simulink model "updated_target_driver_2026_withVariants_MPC_andwlqp"  (R2024b)
settings: Solver=FixedStepDiscrete  StartTime=0.0  StopTime=running_time  FixedStep=dt_s  RelTol=1e-3
values from neighbouring files (symbols this model uses):
  A = gamma_2*gamma_3*Thrust_desired    [force2voltage.m]
  a2_lb = -0.25    [target_driver_setup_2022_Ctrl_V_2_4.m]    (also in target_driver_setup_2022_Ctrl_V_2_4_geometric.m; target_driver_setup_mpc_12msdelay.m; target_driver_setup_mpc_andWLQP.m)
  a2_openloop = 0    [target_driver_setup_2022_Ctrl_V_2_4.m]    (also in target_driver_setup_2022_Ctrl_V_2_4_geometric.m; target_driver_setup_mpc_12msdelay.m; target_driver_setup_mpc_andWLQP.m)
  a2_ub = 0.25    [target_driver_setup_2022_Ctrl_V_2_4.m]    (also in target_driver_setup_2022_Ctrl_V_2_4_geometric.m; target_driver_setup_mpc_12msdelay.m; target_driver_setup_mpc_andWLQP.m)
  att_s = 500    [target_driver_setup_2022_Ctrl_V_2_4.m]    (also in target_driver_setup_2022_Ctrl_V_2_4_geometric.m; target_driver_setup_mpc_12msdelay.m; target_driver_setup_mpc_andWLQP.m)
  b_1_d_desired = [1,0,0]    [target_driver_setup_2022_Ctrl_V_2_4.m]    (also in target_driver_setup_2022_Ctrl_V_2_4_geometric.m; target_driver_setup_mpc_12msdelay.m; target_driver_setup_mpc_andWLQP.m)
  closedloop_flag = 0    [target_driver_setup_2022_Ctrl_V_2_4.m]    (also in target_driver_setup_2022_Ctrl_V_2_4_geometric.m; target_driver_setup_mpc_12msdelay.m; target_driver_setup_mpc_andWLQP.m)
  delay = delay-vicon_sample_cycle/2    [target_driver_setup_2022_Ctrl_V_2_4.m]    (also in target_driver_setup_2022_Ctrl_V_2_4_geometric.m; target_driver_setup_mpc_12msdelay.m; target_driver_setup_mpc_andWLQP.m)
  drv_amp = abs((vleft_p2p-vright_p2p))/2+min(vleft_p2p,vright_p2p)    [Wing_traj_to_Voltage.m]    (also in force2voltage.m; target_driver_setup_2022_Ctrl_V_2_4.m = 150; target_driver_setup_2022_Ctrl_V_2_4_geometric.m = 110; target_driver_setup_mpc_12msdelay.m = 150)
  drv_bias = max_drv_bias    (= 200)    [target_driver_setup_2022_Ctrl_V_2_4.m]    (also in target_driver_setup_2022_Ctrl_V_2_4_geometric.m; target_driver_setup_mpc_12msdelay.m; target_driver_setup_mpc_andWLQP.m)
  drv_pitch_left = vleft_pitch    [Wing_traj_to_Voltage.m]    (also in force2voltage.m = 0; target_driver_setup_2022_Ctrl_V_2_4.m = 9.05; target_driver_setup_2022_Ctrl_V_2_4_geometric.m = 9.05; target_driver_setup_mpc_12msdelay.m = 9.05)
  drv_pitch_right = vright_pitch    [Wing_traj_to_Voltage.m]    (also in force2voltage.m = 0; target_driver_setup_2022_Ctrl_V_2_4.m = 9.05; target_driver_setup_2022_Ctrl_V_2_4_geometric.m = 9.05; target_driver_setup_mpc_12msdelay.m = 9.05)
  drv_roll = (vleft_p2p-vright_p2p)/4    [Wing_traj_to_Voltage.m]    (also in force2voltage.m; target_driver_setup_2022_Ctrl_V_2_4.m = -0.001; target_driver_setup_2022_Ctrl_V_2_4_geometric.m = -0.001; target_driver_setup_mpc_12msdelay.m = -0.001)
  dt_s = 2.0e-4    (= 0.0002)    [target_driver_setup_2022_Ctrl_V_2_4.m]    (also in target_driver_setup_2022_Ctrl_V_2_4_geometric.m; target_driver_setup_mpc_12msdelay.m; target_driver_setup_mpc_andWLQP.m)
  f_fin = f    (= 155)    [target_driver_setup_2022_Ctrl_V_2_4.m]    (also in target_driver_setup_2022_Ctrl_V_2_4_geometric.m; target_driver_setup_mpc_12msdelay.m; target_driver_setup_mpc_andWLQP.m)
  f_int = f    (= 155)    [target_driver_setup_2022_Ctrl_V_2_4.m]    (also in target_driver_setup_2022_Ctrl_V_2_4_geometric.m; target_driver_setup_mpc_12msdelay.m; target_driver_setup_mpc_andWLQP.m)
  g = 9.8    [target_driver_setup_2022_Ctrl_V_2_4.m]    (also in target_driver_setup_2022_Ctrl_V_2_4_geometric.m; target_driver_setup_mpc_12msdelay.m; target_driver_setup_mpc_andWLQP.m; test_full_attitude_mpc.m = 9.81)
  I_moment_vec = [Ixx, Iyy, Izz]    [target_driver_setup_2022_Ctrl_V_2_4.m]    (also in target_driver_setup_2022_Ctrl_V_2_4_geometric.m; target_driver_setup_mpc_12msdelay.m; target_driver_setup_mpc_andWLQP.m)
  k_tau_vec = [k_tau_roll;k_tau_pitch]    [target_driver_setup_2022_Ctrl_V_2_4.m]    (also in target_driver_setup_2022_Ctrl_V_2_4_geometric.m; target_driver_setup_mpc_12msdelay.m; target_driver_setup_mpc_andWLQP.m)
  landing_flag = 0    [target_driver_setup_2022_Ctrl_V_2_4.m]    (also in target_driver_setup_2022_Ctrl_V_2_4_geometric.m; target_driver_setup_mpc_12msdelay.m; target_driver_setup_mpc_andWLQP.m)
  landing_parameter = [start_delay+T,transition_rate, rising_time, falling_time, landing_rising_time, landing_z_decrease, landing_y_decrease, landing_x_decrease]    [target_driver_setup_2022_Ctrl_V_2_4.m]    (also in target_driver_setup_2022_Ctrl_V_2_4_geometric.m; target_driver_setup_mpc_12msdelay.m; target_driver_setup_mpc_andWLQP.m)
  low_bound = -5    [target_driver_setup_2022_Ctrl_V_2_4.m]    (also in target_driver_setup_2022_Ctrl_V_2_4_geometric.m; target_driver_setup_mpc_12msdelay.m = -10; target_driver_setup_mpc_andWLQP.m = -10)
  low_bound_eR = -1.2    [target_driver_setup_2022_Ctrl_V_2_4.m]    (also in target_driver_setup_2022_Ctrl_V_2_4_geometric.m; target_driver_setup_mpc_12msdelay.m; target_driver_setup_mpc_andWLQP.m)
  low_bound_vx = -0.5    [target_driver_setup_2022_Ctrl_V_2_4.m]    (also in target_driver_setup_2022_Ctrl_V_2_4_geometric.m; target_driver_setup_mpc_12msdelay.m; target_driver_setup_mpc_andWLQP.m)
  low_bound_vy = -0.5    [target_driver_setup_2022_Ctrl_V_2_4.m]    (also in target_driver_setup_2022_Ctrl_V_2_4_geometric.m; target_driver_setup_mpc_12msdelay.m; target_driver_setup_mpc_andWLQP.m)
  low_bound_vz = -0.5    [target_driver_setup_2022_Ctrl_V_2_4.m]    (also in target_driver_setup_2022_Ctrl_V_2_4_geometric.m; target_driver_setup_mpc_12msdelay.m; target_driver_setup_mpc_andWLQP.m)
  low_bound_x = -0.1    [target_driver_setup_2022_Ctrl_V_2_4.m]    (also in target_driver_setup_2022_Ctrl_V_2_4_geometric.m; target_driver_setup_mpc_12msdelay.m = -0.6; target_driver_setup_mpc_andWLQP.m = -0.6)
  low_bound_y = -0.06    [target_driver_setup_2022_Ctrl_V_2_4.m]    (also in target_driver_setup_2022_Ctrl_V_2_4_geometric.m; target_driver_setup_mpc_12msdelay.m = -0.6; target_driver_setup_mpc_andWLQP.m = -0.6)
  low_bound_z = -0.04    [target_driver_setup_2022_Ctrl_V_2_4.m]    (also in target_driver_setup_2022_Ctrl_V_2_4_geometric.m; target_driver_setup_mpc_12msdelay.m = -0.1; target_driver_setup_mpc_andWLQP.m = -0.1)
  m = t <= t_zoom    [plot_roll_torque_cmd_vs_actual.m]    (also in plot_roll_torque_cmd_vs_actual_flightlog.m = t >= t0 & t <= t1; target_driver_setup_2022_Ctrl_V_2_4.m = 8.5655e-05; target_driver_setup_2022_Ctrl_V_2_4_geometric.m = 8.5655e-05; target_driver_setup_mpc_12msdelay.m = 8.5655e-05)
  params_vec = [params_opt.delta_1, params_opt.delta_2, params_opt.delta_3,      params_opt.gamma_1, params_opt.gamma_2_1, params_opt.gamma_3,      params_opt.eta, params_opt.nu, params_opt.mu]'    [force2voltage_tuningSandbox.m]    (also in target_driver_setup_2022_Ctrl_V_2_4.m = [params_opt.delta_1, params_opt.delta_2, params_opt.delta_3,; target_driver_setup_2022_Ctrl_V_2_4_geometric.m = [params_opt.delta_1, params_opt.delta_2, params_opt.delta_3,; target_driver_setup_mpc_12msdelay.m = [params_opt.delta_1, params_opt.delta_2, params_opt.delta_3,; target_driver_setup_mpc_andWLQP.m = [params_opt.delta_1, params_opt.delta_2, params_opt.delta_3,)
  phase = 0    [target_driver_setup_2022_Ctrl_V_2_4.m]    (also in target_driver_setup_2022_Ctrl_V_2_4_geometric.m; target_driver_setup_mpc_12msdelay.m; target_driver_setup_mpc_andWLQP.m)
  r_desired = [default_x, default_y,z_desired]    [target_driver_setup_2022_Ctrl_V_2_4.m]    (also in target_driver_setup_2022_Ctrl_V_2_4_geometric.m; target_driver_setup_mpc_12msdelay.m; target_driver_setup_mpc_andWLQP.m)
  roll_offset_angle = 0    [target_driver_setup_2022_Ctrl_V_2_4.m]    (also in target_driver_setup_2022_Ctrl_V_2_4_geometric.m; target_driver_setup_mpc_12msdelay.m; target_driver_setup_mpc_andWLQP.m)
  running_time = start_delay+T    (= 10)    [target_driver_setup_2022_Ctrl_V_2_4.m]    (also in target_driver_setup_2022_Ctrl_V_2_4_geometric.m; target_driver_setup_mpc_12msdelay.m = 0.5; target_driver_setup_mpc_andWLQP.m)
  running_time_control = start_delay_control+T+0.0    (= 10)    [target_driver_setup_2022_Ctrl_V_2_4.m]    (also in target_driver_setup_2022_Ctrl_V_2_4_geometric.m; target_driver_setup_mpc_12msdelay.m = 0.5; target_driver_setup_mpc_andWLQP.m)
  sampling_f = 1/dt_s    (= 5000)    [target_driver_setup_2022_Ctrl_V_2_4.m]    (also in target_driver_setup_2022_Ctrl_V_2_4_geometric.m; target_driver_setup_mpc_12msdelay.m; target_driver_setup_mpc_andWLQP.m)
  start_delay = 0.0    (= 0)    [target_driver_setup_2022_Ctrl_V_2_4.m]    (also in target_driver_setup_2022_Ctrl_V_2_4_geometric.m; target_driver_setup_mpc_12msdelay.m; target_driver_setup_mpc_andWLQP.m)
  start_delay_control = start_delay + ramp_delay    (= 0)    [target_driver_setup_2022_Ctrl_V_2_4.m]    (also in target_driver_setup_2022_Ctrl_V_2_4_geometric.m; target_driver_setup_mpc_12msdelay.m; target_driver_setup_mpc_andWLQP.m)
  T = 10    [target_driver_setup_2022_Ctrl_V_2_4.m]    (also in target_driver_setup_2022_Ctrl_V_2_4_geometric.m; target_driver_setup_mpc_12msdelay.m = 0.5; target_driver_setup_mpc_andWLQP.m; test_full_attitude_mpc.m = T0 + nu(1))
  task_flag = 0    [target_driver_setup_2022_Ctrl_V_2_4.m]    (also in target_driver_setup_2022_Ctrl_V_2_4_geometric.m; target_driver_setup_mpc_12msdelay.m; target_driver_setup_mpc_andWLQP.m)
  task_parameter = [radius_ref, frequency_ref, radius_ratio, lissajous_ratio, lissajous_delta, lissajous_amplitude_ratio,z_radius_ratio]    [target_driver_setup_2022_Ctrl_V_2_4.m]    (also in target_driver_setup_2022_Ctrl_V_2_4_geometric.m; target_driver_setup_mpc_12msdelay.m; target_driver_setup_mpc_andWLQP.m)
  upp_bound = 5    [target_driver_setup_2022_Ctrl_V_2_4.m]    (also in target_driver_setup_2022_Ctrl_V_2_4_geometric.m; target_driver_setup_mpc_12msdelay.m = 10; target_driver_setup_mpc_andWLQP.m = 10)
  upp_bound_eR = 1.2    [target_driver_setup_2022_Ctrl_V_2_4.m]    (also in target_driver_setup_2022_Ctrl_V_2_4_geometric.m; target_driver_setup_mpc_12msdelay.m; target_driver_setup_mpc_andWLQP.m)
  upp_bound_vx = 0.5    [target_driver_setup_2022_Ctrl_V_2_4.m]    (also in target_driver_setup_2022_Ctrl_V_2_4_geometric.m; target_driver_setup_mpc_12msdelay.m; target_driver_setup_mpc_andWLQP.m)
  upp_bound_vy = 0.5    [target_driver_setup_2022_Ctrl_V_2_4.m]    (also in target_driver_setup_2022_Ctrl_V_2_4_geometric.m; target_driver_setup_mpc_12msdelay.m; target_driver_setup_mpc_andWLQP.m)
  upp_bound_vz = 0.5    [target_driver_setup_2022_Ctrl_V_2_4.m]    (also in target_driver_setup_2022_Ctrl_V_2_4_geometric.m; target_driver_setup_mpc_12msdelay.m; target_driver_setup_mpc_andWLQP.m)
  upp_bound_x = 0.1    [target_driver_setup_2022_Ctrl_V_2_4.m]    (also in target_driver_setup_2022_Ctrl_V_2_4_geometric.m; target_driver_setup_mpc_12msdelay.m = 0.6; target_driver_setup_mpc_andWLQP.m = 0.6)
  upp_bound_y = 0.06    [target_driver_setup_2022_Ctrl_V_2_4.m]    (also in target_driver_setup_2022_Ctrl_V_2_4_geometric.m; target_driver_setup_mpc_12msdelay.m = 0.6; target_driver_setup_mpc_andWLQP.m = 0.6)
  upp_bound_z = 0.04    [target_driver_setup_2022_Ctrl_V_2_4.m]    (also in target_driver_setup_2022_Ctrl_V_2_4_geometric.m; target_driver_setup_mpc_12msdelay.m = 0.1; target_driver_setup_mpc_andWLQP.m = 0.1)
  weights_vec = [ws; wds; wpr_xy;wpr_z; wpf; wvr_xy; wvr_z ... (first row only)    [target_driver_setup_2022_Ctrl_V_2_4.m]    (also in target_driver_setup_2022_Ctrl_V_2_4_geometric.m; target_driver_setup_mpc_12msdelay.m; target_driver_setup_mpc_andWLQP.m)
undefined symbols (not defined in the file or in its folder): Com1, ctrl_Ts, DiscIntNeverNeededParam, dspblkCoreblockFVToolHelper, gcbh, left_mapping, left_mapping_F_to_Phi, lp_den, lp_num, none, right_mapping, right_mapping_F_to_Phi, vlp_den, vlp_num
libraries: simulink x18, xpcseriallib x2, cstblocks x1, xpcnilib x1, xpcutilitieslib x1
(part 2 of 6)

== system updated_target_driver_2026_withVariants_MPC_andwlqp/Variant Subsystem/Experimental ==
  EnableSignal : Inport
  frequency (hz) : Inport  Port=2
  Amplitude : Inport  Port=3
  PitchBias V (left) : Inport  Port=4
  RollBias V : Inport  Port=5
  PitchBias V (right) : Inport  Port=6
  a2 : Inport  Port=7
  Bias_v : Inport  Port=8
  Phase (deg) : Inport  Port=9
  In10 : Inport  Port=10
  PCI-6259 DA1 : xpcnilib/D//A/M Series/PCI-6259 DA  channel=[1:4]  range=[10,5, 10, 10]  reset=[1 1 1 1]  initValue=[0 0 0 0]  sampletime=-1  slot=-1
      settings: SourceProductName=Simulink Real-Time
  Vicon Measurements1 : Subsystem
  signal generator a3 : Subsystem
  bias2 : Outport
  LW signal : Outport  Port=2
  RW signal : Outport  Port=3
  X (m) : Outport  Port=4
  Y (m) : Outport  Port=5
  Z (m) : Outport  Port=6
  alpha (radians) : Outport  Port=7
  beta (radians) : Outport  Port=8
  gamma (radians) : Outport  Port=9
  wires:
  Vicon Measurements1/2(Y (m)) -> Y (m)/1
  PitchBias V (right)/1 -> signal generator a3/8(PitchBias V (right))
  a2/1 -> signal generator a3/9(a2)
  Phase (deg)/1 -> signal generator a3/7(Phase (deg))
  Vicon Measurements1/4(alpha (radians)) -> alpha (radians)/1
  frequency (hz)/1 -> signal generator a3/3(frequency (hz))
  RollBias V/1 -> signal generator a3/6(RollBias V)
  Bias_v/1 -> signal generator a3/2(Bias_v)
  Vicon Measurements1/6(gamma (radians)) -> gamma (radians)/1
  Amplitude/1 -> signal generator a3/4(Amplitude)
  Vicon Measurements1/5(beta (radians)) -> beta (radians)/1
  signal generator a3/3(D2A DriveSignal 2) -> RW signal/1, PCI-6259 DA1/3
  signal generator a3/1(Bias_D2A) -> bias2/1, PCI-6259 DA1/1
  Vicon Measurements1/1(X (m)) -> X (m)/1
  Vicon Measurements1/3(Z (m)) -> Z (m)/1
  In10/1 -> PCI-6259 DA1/4
  PitchBias V (left)/1 -> signal generator a3/5(PitchBias V (left))
  EnableSignal/1 -> signal generator a3/1(EnableSignal)
  signal generator a3/2(D2A DriveSignal 1) -> LW signal/1, PCI-6259 DA1/2

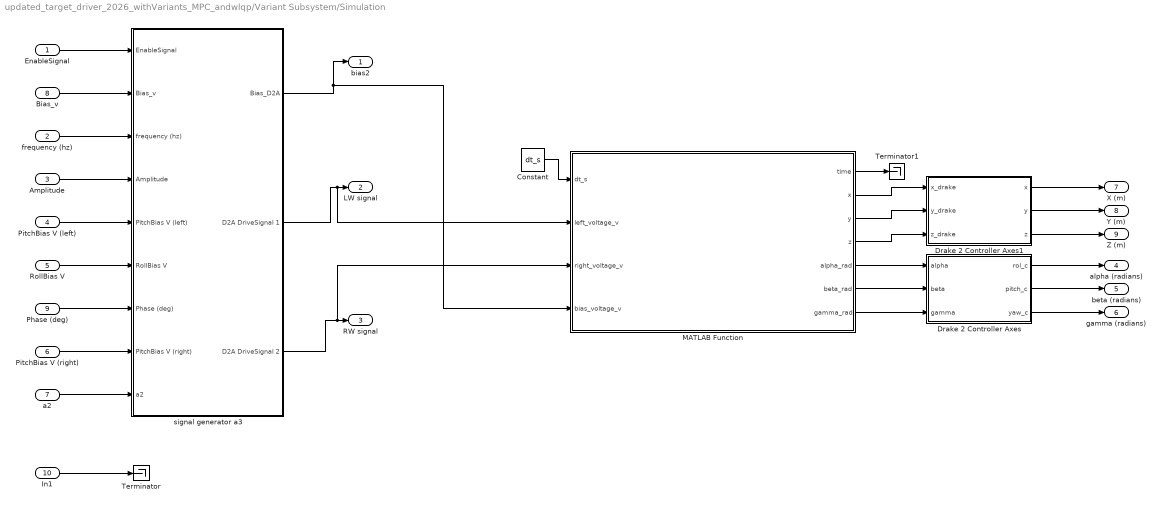
== system updated_target_driver_2026_withVariants_MPC_andwlqp/Variant Subsystem/Simulation ==
  EnableSignal : Inport
  frequency (hz) : Inport  Port=2
  Amplitude : Inport  Port=3
  PitchBias V (left) : Inport  Port=4
  RollBias V : Inport  Port=5
  PitchBias V (right) : Inport  Port=6
  a2 : Inport  Port=7
  Bias_v : Inport  Port=8
  Phase (deg) : Inport  Port=9
  In1 : Inport  Port=10
  Constant : Constant  Value=dt_s
  Drake 2 Controller Axes : MATLAB Function  TreatAsAtomicUnit=on
  Drake 2 Controller Axes1 : MATLAB Function  TreatAsAtomicUnit=on
  MATLAB Function : MATLAB Function  TreatAsAtomicUnit=on  VariantControl=Choice_1
  Terminator : Terminator
  Terminator1 : Terminator
  signal generator a3 : Subsystem
  bias2 : Outport
  LW signal : Outport  Port=2
  RW signal : Outport  Port=3
  alpha (radians) : Outport  Port=4
  beta (radians) : Outport  Port=5
  gamma (radians) : Outport  Port=6
  X (m) : Outport  Port=7
  Y (m) : Outport  Port=8
  Z (m) : Outport  Port=9
  wires:
  signal generator a3/1(Bias_D2A) -> bias2/1, MATLAB Function/4(bias_voltage_v)
  Constant/1 -> MATLAB Function/1(dt_s)
  signal generator a3/3(D2A DriveSignal 2) -> MATLAB Function/3(right_voltage_v), RW signal/1
  a2/1 -> signal generator a3/9(a2)
  PitchBias V (left)/1 -> signal generator a3/5(PitchBias V (left))
  Amplitude/1 -> signal generator a3/4(Amplitude)
  Bias_v/1 -> signal generator a3/2(Bias_v)
  PitchBias V (right)/1 -> signal generator a3/8(PitchBias V (right))
  RollBias V/1 -> signal generator a3/6(RollBias V)
  Phase (deg)/1 -> signal generator a3/7(Phase (deg))
  frequency (hz)/1 -> signal generator a3/3(frequency (hz))
  EnableSignal/1 -> signal generator a3/1(EnableSignal)
  In1/1 -> Terminator/1
  MATLAB Function/1(time) -> Terminator1/1
  MATLAB Function/4(z) -> Drake 2 Controller Axes1/3(z_drake)
  MATLAB Function/3(y) -> Drake 2 Controller Axes1/2(y_drake)
  MATLAB Function/2(x) -> Drake 2 Controller Axes1/1(x_drake)
  MATLAB Function/5(alpha_rad) -> Drake 2 Controller Axes/1(alpha)
  MATLAB Function/6(beta_rad) -> Drake 2 Controller Axes/2(beta)
  MATLAB Function/7(gamma_rad) -> Drake 2 Controller Axes/3(gamma)
  Drake 2 Controller Axes/1(rol_c) -> alpha (radians)/1
  Drake 2 Controller Axes/2(pitch_c) -> beta (radians)/1
  Drake 2 Controller Axes/3(yaw_c) -> gamma (radians)/1
  Drake 2 Controller Axes1/2(y) -> Y (m)/1
  Drake 2 Controller Axes1/1(x) -> X (m)/1
  Drake 2 Controller Axes1/3(z) -> Z (m)/1
  signal generator a3/2(D2A DriveSignal 1) -> MATLAB Function/2(left_voltage_v), LW signal/1

== system updated_target_driver_2026_withVariants_MPC_andwlqp/Vicon Post Processing1/Raw rotation matrix ==
  alpha : Inport
  beta : Inport  Port=2
  gamma : Inport  Port=3
  Mux : Mux  Inputs=9
  Rotation Matrix : Subsystem
  R : Outport
  wires:
  alpha/1 -> Rotation Matrix/1(alpha)
  beta/1 -> Rotation Matrix/2(beta)
  gamma/1 -> Rotation Matrix/3(gamma)
  Mux/1 -> R/1
  Rotation Matrix/1(R11) -> Mux/1
  Rotation Matrix/2(R12) -> Mux/2
  Rotation Matrix/3(R13) -> Mux/3
  Rotation Matrix/4(R21) -> Mux/4
  Rotation Matrix/5(R22) -> Mux/5
  Rotation Matrix/6(R23) -> Mux/6
  Rotation Matrix/7(R31) -> Mux/7
  Rotation Matrix/8(R32) -> Mux/8
  Rotation Matrix/9(R33) -> Mux/9

== system updated_target_driver_2026_withVariants_MPC_andwlqp/Vicon Post Processing1/Vicon Validity check ==
  "Rotation Matrix " : Inport
  Compare To Zero2 : simulink/Logic and Bit Operations/Compare To Zero  relop===  OutDataTypeStr=uint8
  Constant : Constant
  Data Type Conversion1 : DataTypeConversion  OutDataTypeStr=double  SaturateOnIntegerOverflow=off  RndMeth=Floor
  Delay : Delay  DelayLength=1  InitialCondition=0
  Delay2 : Delay  DelayLength=1  InitialCondition=0
  MATLAB Function3 : MATLAB Function  TreatAsAtomicUnit=on
  SaturatingRamp : DiscreteIntegrator  gainval=sampling_f  ExternalReset=falling  SampleTime=-1  UpperSaturationLimit=1  LowerSaturationLimit=0  ICPrevOutput=DiscIntNeverNeededParam  ICPrevScaledInput=DiscIntNeverNeededParam
  Variant Subsystem1 : Subsystem  Variant=on
  type conv : DataTypeConversion  OutDataTypeStr=double  SaturateOnIntegerOverflow=off  RndMeth=Floor
  "Vicon Update flag " : Outport
  Vicon Count : Outport  Port=2
  wires:
  Delay/1 -> MATLAB Function3/1(R_prev)
  SaturatingRamp/1 -> Data Type Conversion1/1
  type conv/1 -> SaturatingRamp/2
  Constant/1 -> SaturatingRamp/1
  Compare To Zero2/1 -> type conv/1
  "Rotation Matrix "/1 -> MATLAB Function3/2(R_cur), Delay/1
  Delay2/1 -> Vicon Count/1
  Data Type Conversion1/1 -> "Vicon Update flag "/1, Delay2/1
  MATLAB Function3/1(y) -> Variant Subsystem1/1(In1)
  Variant Subsystem1/1(Out1) -> Compare To Zero2/1

== system updated_target_driver_2026_withVariants_MPC_andwlqp/Desired attitude and normalized error/Geometric derivative for Rd in SO(3)/filtered derivative1 ==
  In1 : Inport
  low pass3 : DiscreteTransferFcn  Numerator=vlp_num  Denominator=vlp_den
  Out1 : Outport
  wires:
  low pass3/1 -> Out1/1
  In1/1 -> low pass3/1

== system updated_target_driver_2026_withVariants_MPC_andwlqp/Desired attitude and normalized error/Geometric derivative for Rd in SO(3)/filtered derivative5 ==
  In1 : Inport
  low pass3 : DiscreteTransferFcn  Numerator=lp_num  Denominator=lp_den
  Out1 : Outport
  wires:
  low pass3/1 -> Out1/1
  In1/1 -> low pass3/1

== system updated_target_driver_2026_withVariants_MPC_andwlqp/Desired attitude and normalized error/Variant Subsystem/saturated normalized error observation ==
  p : Inport
  v : Inport  Port=2
  R : Inport  Port=3
  omega : Inport  Port=4
  "omega_desired " : Inport  Port=5
  R_desired : Inport  Port=6
  r_desired : Inport  Port=7
  "v_desired " : Inport  Port=8
  "Saturated angular velocity eOmega " : Subsystem
  Saturated normalized eR : Subsystem
  "saturated normalized altitude error " : Subsystem
  "Normalized omega error " : Outport
  Normalized eR : Outport  Port=2
  "Normalized position error " : Outport  Port=3
  Normalized velocity error : Outport  Port=4
  wires:
  omega/1 -> "Saturated angular velocity eOmega "/1(omega)
  v/1 -> "saturated normalized altitude error "/1(averaged velocity)
  p/1 -> "saturated normalized altitude error "/2(averaged position)
  Saturated normalized eR/1(normalized eR) -> Normalized eR/1
  R/1 -> "Saturated angular velocity eOmega "/3(R_cur), Saturated normalized eR/1(Current averaged rotation M)
  R_desired/1 -> "Saturated angular velocity eOmega "/4(R_desired), Saturated normalized eR/2(R_desired)
  "Saturated angular velocity eOmega "/1(Normalized angular velocity) -> "Normalized omega error "/1
  "omega_desired "/1 -> "Saturated angular velocity eOmega "/2("omega_desired ")
  "saturated normalized altitude error "/1(Position error) -> "Normalized position error "/1
  "saturated normalized altitude error "/2(velocity_error) -> Normalized velocity error/1
  "v_desired "/1 -> "saturated normalized altitude error "/4(v_desired)
  r_desired/1 -> "saturated normalized altitude error "/3("r_desired ")

== system updated_target_driver_2026_withVariants_MPC_andwlqp/Desired attitude and normalized error/Variant Subsystem/unsaturated normalized error observation1 ==
  p : Inport
  v : Inport  Port=2
  R : Inport  Port=3
  omega : Inport  Port=4
  "omega_desired " : Inport  Port=5
  R_desired : Inport  Port=6
  r_desired : Inport  Port=7
  "v_desired " : Inport  Port=8
  "Saturated angular velocity eOmega " : Subsystem
  Saturated normalized eR : Subsystem
  "saturated normalized altitude error " : Subsystem
  "Normalized omega error " : Outport
  Normalized eR : Outport  Port=2
  "Normalized position error " : Outport  Port=3
  Normalized velocity error : Outport  Port=4
  wires:
  omega/1 -> "Saturated angular velocity eOmega "/1(omega)
  v/1 -> "saturated normalized altitude error "/1(averaged velocity)
  p/1 -> "saturated normalized altitude error "/2(averaged position)
  Saturated normalized eR/1(normalized eR) -> Normalized eR/1
  R/1 -> "Saturated angular velocity eOmega "/3(R_cur), Saturated normalized eR/1(Current averaged rotation M)
  R_desired/1 -> "Saturated angular velocity eOmega "/4(R_desired), Saturated normalized eR/2(R_desired)
  "Saturated angular velocity eOmega "/1(Normalized angular velocity) -> "Normalized omega error "/1
  "omega_desired "/1 -> "Saturated angular velocity eOmega "/2("omega_desired ")
  "saturated normalized altitude error "/1(Position error) -> "Normalized position error "/1
  "saturated normalized altitude error "/2(velocity_error) -> Normalized velocity error/1
  "v_desired "/1 -> "saturated normalized altitude error "/4(v_desired)
  r_desired/1 -> "saturated normalized altitude error "/3("r_desired ")

== system updated_target_driver_2026_withVariants_MPC_andwlqp/Force to voltage/Control Mode/Force_to_Voltage1 ==
  note: Mapping from desired Thrust/Torque to Wing traj to Voltage mapping
      |
      | Patrick Hyun 2021 Apr
  note: a2: second-harmonic coefficient
      | Franklin Ho Jun 2026
  "Thrust_desired " : Inport
  Roll_torque_desired : Inport  Port=2
  Pitch_torque_desired : Inport  Port=3
  Yaw_torque_desired : Inport  Port=4
  A : Constant  Commented=on  Value=A
  Desired_Force_to_Voltage : MATLAB Function  TreatAsAtomicUnit=on
  "Force to Trajectory " : MATLAB Function  Commented=on  TreatAsAtomicUnit=on
  "Trajectory to Voltage Input " : MATLAB Function  Commented=on  TreatAsAtomicUnit=on
  left_mapping : Constant  Commented=on  Value=left_mapping
  left_mapping_F_to_Phi : Constant  Commented=on  Value=left_mapping_F_to_Phi
  params_vec : Constant  Value=params_vec
  right_mapping1 : Constant  Commented=on  Value=right_mapping
  right_mapping_F_to_Phi : Constant  Commented=on  Value=right_mapping_F_to_Phi
  drv_amp : Outport
  drv_pitch_left : Outport  Port=2
  drv_pitch_right : Outport  Port=3
  drv_roll : Outport  Port=4
  a2 : Outport  Port=5
  wires:
  left_mapping/1 -> "Trajectory to Voltage Input "/4(left_mapping)
  right_mapping1/1 -> "Trajectory to Voltage Input "/5(right_mapping)
  A/1 -> "Force to Trajectory "/6(A)
  "Force to Trajectory "/1(Phi_left_p2p_desired) -> "Trajectory to Voltage Input "/1(Phi_left_p2p_command)
  "Force to Trajectory "/2(Phi_right_p2p_desired) -> "Trajectory to Voltage Input "/2(Phi_right_p2p_command)
  "Force to Trajectory "/3(Phi_pitch_desired) -> "Trajectory to Voltage Input "/3(Phi_pitch_command)
  left_mapping_F_to_Phi/1 -> "Force to Trajectory "/4(left_mapping_F_to_Phi)
  right_mapping_F_to_Phi/1 -> "Force to Trajectory "/5(right_mapping_F_to_Phi)
  Desired_Force_to_Voltage/4(drv_pitch_right) -> drv_pitch_right/1
  Desired_Force_to_Voltage/3(drv_pitch_left) -> drv_pitch_left/1
  Desired_Force_to_Voltage/2(drv_roll) -> drv_roll/1
  Desired_Force_to_Voltage/1(drv_amp) -> drv_amp/1
  "Thrust_desired "/1 -> Desired_Force_to_Voltage/1(Thrust_desired)
  Pitch_torque_desired/1 -> Desired_Force_to_Voltage/3(Pitch_torque_desired)
  Yaw_torque_desired/1 -> Desired_Force_to_Voltage/4(Yaw_torque_desired)
  params_vec/1 -> Desired_Force_to_Voltage/5(params_vec)
  Desired_Force_to_Voltage/5(a2_coeff) -> a2/1
  Roll_torque_desired/1 -> Desired_Force_to_Voltage/2(Roll_torque_desired)

== system updated_target_driver_2026_withVariants_MPC_andwlqp/Force to voltage/Replay Mode/Force_to_Voltage1 ==
  note: a2: second-harmonic coefficient
      | Franklin Ho Jun 2026
  note: Mapping from desired Thrust/Torque to Wing traj to Voltage mapping
      |
      | Patrick Hyun 2021 Apr
  "Thrust_desired " : Inport
  Roll_torque_desired : Inport  Port=2
  Pitch_torque_desired : Inport  Port=3
  Yaw_torque_desired : Inport  Port=4
  A : Constant  Commented=on  Value=A
  Desired_Force_to_Voltage : MATLAB Function  TreatAsAtomicUnit=on
  "Force to Trajectory " : MATLAB Function  Commented=on  TreatAsAtomicUnit=on
  Saturation : Saturate  UpperLimit=a2_ub  LowerLimit=a2_lb
  "Trajectory to Voltage Input " : MATLAB Function  Commented=on  TreatAsAtomicUnit=on
  left_mapping : Constant  Commented=on  Value=left_mapping
  left_mapping_F_to_Phi : Constant  Commented=on  Value=left_mapping_F_to_Phi
  params_vec : Constant  Value=params_vec
  right_mapping1 : Constant  Commented=on  Value=right_mapping
  right_mapping_F_to_Phi : Constant  Commented=on  Value=right_mapping_F_to_Phi
  drv_amp : Outport
  drv_pitch_left : Outport  Port=2
  drv_pitch_right : Outport  Port=3
  drv_roll : Outport  Port=4
  a2 : Outport  Port=5
  wires:
  Roll_torque_desired/1 -> Desired_Force_to_Voltage/2(Roll_torque_desired)
  Saturation/1 -> a2/1
  Desired_Force_to_Voltage/5(a2_coeff) -> Saturation/1
  params_vec/1 -> Desired_Force_to_Voltage/5(params_vec)
  Yaw_torque_desired/1 -> Desired_Force_to_Voltage/4(Yaw_torque_desired)
  Pitch_torque_desired/1 -> Desired_Force_to_Voltage/3(Pitch_torque_desired)
  "Thrust_desired "/1 -> Desired_Force_to_Voltage/1(Thrust_desired)
  Desired_Force_to_Voltage/1(drv_amp) -> drv_amp/1
  Desired_Force_to_Voltage/2(drv_roll) -> drv_roll/1
  Desired_Force_to_Voltage/3(drv_pitch_left) -> drv_pitch_left/1
  Desired_Force_to_Voltage/4(drv_pitch_right) -> drv_pitch_right/1
  right_mapping_F_to_Phi/1 -> "Force to Trajectory "/5(right_mapping_F_to_Phi)
  left_mapping_F_to_Phi/1 -> "Force to Trajectory "/4(left_mapping_F_to_Phi)
  "Force to Trajectory "/3(Phi_pitch_desired) -> "Trajectory to Voltage Input "/3(Phi_pitch_command)
  "Force to Trajectory "/2(Phi_right_p2p_desired) -> "Trajectory to Voltage Input "/2(Phi_right_p2p_command)
  "Force to Trajectory "/1(Phi_left_p2p_desired) -> "Trajectory to Voltage Input "/1(Phi_left_p2p_command)
  A/1 -> "Force to Trajectory "/6(A)
  right_mapping1/1 -> "Trajectory to Voltage Input "/5(right_mapping)
  left_mapping/1 -> "Trajectory to Voltage Input "/4(left_mapping)

== system updated_target_driver_2026_withVariants_MPC_andwlqp/Observer for averaged system1/Attitude Observer/Geometric Averaging Rotation Matix ==
  note: Geometric mean in SO(3)
      | 1) Output the Geometric average over one cycle (n=4 samples: 500Hz vicon sampling and 160Hz flapping signal)
      |
      | Patrick 2021 Mar
  Vicon Update flag : Inport
  Current Rotation : Inport  Port=2
  Averaged quaternion : MATLAB Function  TreatAsAtomicUnit=on
  Delay6 : Delay  DelayLength=1  InitialCondition=0
  Demux3 : Demux
  Demux4 : Demux
  Geometric Averaging Rotation M : Subsystem
  Mux3 : Mux
  Mux4 : Mux
  Raw quaternion : MATLAB Function  TreatAsAtomicUnit=on
  Averaged quaternion output : Outport
  "Averaged Rotation Matrix " : Outport  Port=2
  "Raw quaternion output " : Outport  Port=3
  Previous Averaged Rotation Matrix : Outport  Port=4
  wires:
  Raw quaternion/1(quat) -> Demux4/1
  Demux4/3 -> Mux4/3
  Demux4/4 -> Mux4/4
  Demux4/1 -> Mux4/1
  Demux4/2 -> Mux4/2
  Mux4/1 -> "Raw quaternion output "/1
  Vicon Update flag/1 -> Geometric Averaging Rotation M/2(Vicon Update)
  Current Rotation/1 -> Raw quaternion/1(R), Geometric Averaging Rotation M/1("Current Rotation ")
  Mux3/1 -> Averaged quaternion output/1
  Demux3/4 -> Mux3/4
  Averaged quaternion/1(quat) -> Demux3/1
  Demux3/3 -> Mux3/3
  Geometric Averaging Rotation M/1(Averaged Rotation Matrix) -> Delay6/1, Averaged quaternion/1(R), "Averaged Rotation Matrix "/1
  Demux3/2 -> Mux3/2
  Demux3/1 -> Mux3/1
  Delay6/1 -> Geometric Averaging Rotation M/3("Previous Averaged Rotation "), Previous Averaged Rotation Matrix/1

== system updated_target_driver_2026_withVariants_MPC_andwlqp/Observer for averaged system1/Attitude Observer/Geometric derivative in SO(3) ==
  note: First order geometric derivative in SO(3)
      | Patrick 2021 Mar
  Previous Averaged Rotation M : Inport
  Vicon Count : Inport  Port=2
  Current Averaged Rotation M : Inport  Port=3
  "Vicon Update Flag " : Inport  Port=4
  Constant : Constant  Value=sampling_f
  Demux2 : Demux  Outputs=3
  "First order geometric derivative in SO(3) " : MATLAB Function  TreatAsAtomicUnit=on
  Mux2 : Mux  Inputs=3
  Previous Omega : Delay  DelayLength=1  InitialCondition=0
  filtered derivative5 : Subsystem
  Filtered Geometric derivative in SO(3) : Outport
  wires:
  Previous Omega/1 -> "First order geometric derivative in SO(3) "/3(omega_prev)
  Previous Averaged Rotation M/1 -> "First order geometric derivative in SO(3) "/1(R_prev)
  Demux2/1 -> Mux2/1
  Demux2/2 -> Mux2/2
  filtered derivative5/1(Out1) -> Demux2/1
  Mux2/1 -> Filtered Geometric derivative in SO(3)/1
  "First order geometric derivative in SO(3) "/1(omega) -> Previous Omega/1, filtered derivative5/1(In1)
  Demux2/3 -> Mux2/3
  "Vicon Update Flag "/1 -> "First order geometric derivative in SO(3) "/4(update)
  Current Averaged Rotation M/1 -> "First order geometric derivative in SO(3) "/2(R_cur)
  Vicon Count/1 -> "First order geometric derivative in SO(3) "/5(count)
  Constant/1 -> "First order geometric derivative in SO(3) "/6(sampling_f)

== system updated_target_driver_2026_withVariants_MPC_andwlqp/Observer for averaged system1/Euler derivative & filtered angular velocity /filtered derivative ==
  In1 : Inport
  att_s : Gain  Gain=att_s
  filtered derivative : simulink/Discrete/Transfer Fcn Lead or Lag  PoleZ=k_da  ZeroZ=1  ICPrevOutput=0.0  ICPrevInput=0.0  DoSatur=off
  low pass3 : DiscreteTransferFcn  Numerator=lp_num  Denominator=lp_den
  Out1 : Outport
  wires:
  att_s/1 -> filtered derivative/1
  In1/1 -> att_s/1
  low pass3/1 -> Out1/1
  filtered derivative/1 -> low pass3/1

== system updated_target_driver_2026_withVariants_MPC_andwlqp/Observer for averaged system1/Position Observer/LowPassFilter1 ==
  In1 : Inport
  low pass3 : DiscreteTransferFcn  Numerator=lp_num  Denominator=lp_den
  Out1 : Outport
  wires:
  low pass3/1 -> Out1/1
  In1/1 -> low pass3/1

== system updated_target_driver_2026_withVariants_MPC_andwlqp/Observer for averaged system1/Position Observer/LowPassFilter2 ==
  In1 : Inport
  low pass3 : DiscreteTransferFcn  Numerator=lp_num  Denominator=lp_den
  Out1 : Outport
  wires:
  low pass3/1 -> Out1/1
  In1/1 -> low pass3/1

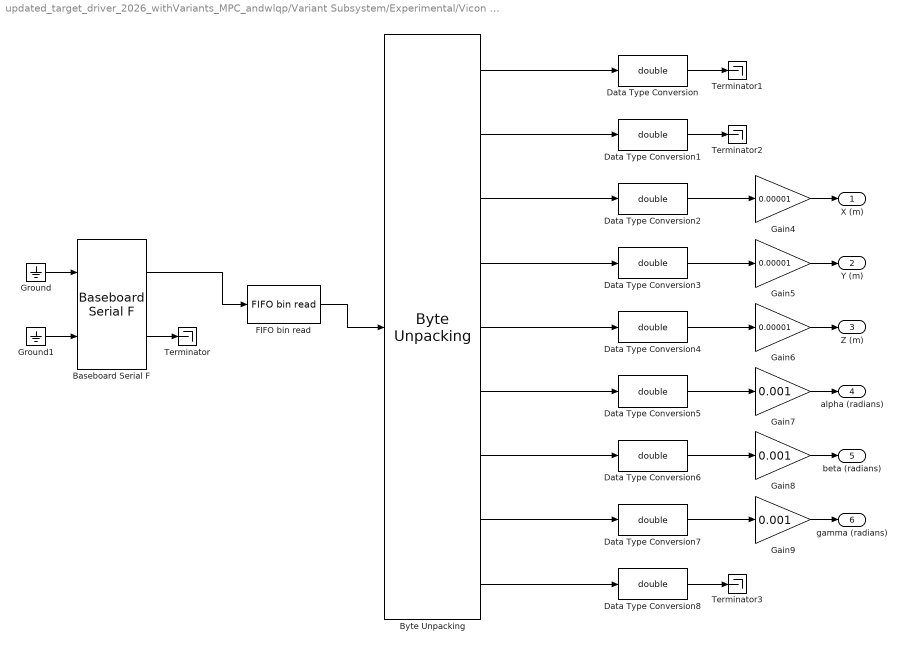
== system updated_target_driver_2026_withVariants_MPC_andwlqp/Variant Subsystem/Experimental/Vicon Measurements1 ==
  Baseboard Serial F : xpcseriallib/Mainboard/Baseboard Serial F  group=FIFO Setup  port=1  irqnum=4  saddr1=0x3f8  saddr2=0x3e8  config=Com1/none  baud1=115200  parity1=None  ndata1=8  nstop1=1  fifomode1=16 deep  rlevel1=half full  automode1=on  xmtfifosize1=1024  xmtdatatype1=8 bit int null terminated  rcvfifosize1=1024  baud2=115200  parity2=None  ndata2=8  nstop2=1  fifomode2=16 deep  rlevel2=half full  automode2=off  xmtfifosize2=1024  xmtdatatype2=8 bit uint null terminated  rcvfifosize2=1024
      settings: SourceProductName=Simulink Real-Time
  "Byte Unpacking " : xpcutilitieslib/Byte Unpacking   MaskUnpackedDataTypes={'uint8','int16','int16','int16','int16','int16','int16','int16','uint8'}  MaskUnpackedDataSizes={[1] [1] [1] [1] [1] [1] [1] [1] [1]}  MaskAlignment=1
      settings: SourceProductName=Simulink Real-Time
  Data Type Conversion{,1..8} (9 alike) : DataTypeConversion  OutDataTypeStr=double  SaturateOnIntegerOverflow=off  RndMeth=Floor
  "FIFO bin read " : xpcseriallib/FIFO bin read   header=[128,127,127]  lengths=[15]  hold=Hold last output if no new data  enable=off  maxsize=15  outputtype=8 bit uint null terminated  sampletime=0.0001
      settings: SourceProductName=Simulink Real-Time
  Gain4 : Gain  Gain=0.00001
  Gain5 : Gain  Gain=0.00001
  Gain6 : Gain  Gain=0.00001
  Gain7 : Gain  Gain=0.001
  Gain8 : Gain  Gain=0.001
  Gain9 : Gain  Gain=0.001
  Ground : Ground
  Ground1 : Ground
  Terminator{,1..3} (4 alike) : Terminator
  X (m) : Outport
  Y (m) : Outport  Port=2
  Z (m) : Outport  Port=3
  alpha (radians) : Outport  Port=4
  beta (radians) : Outport  Port=5
  gamma (radians) : Outport  Port=6
  wires:
  Baseboard Serial F/1 -> "FIFO bin read "/1
  Baseboard Serial F/2 -> Terminator/1
  Ground1/1 -> Baseboard Serial F/2
  Ground/1 -> Baseboard Serial F/1
  "Byte Unpacking "/1 -> Data Type Conversion/1
  "Byte Unpacking "/2 -> Data Type Conversion1/1
  "Byte Unpacking "/3 -> Data Type Conversion2/1
  "Byte Unpacking "/4 -> Data Type Conversion3/1
  "FIFO bin read "/1 -> "Byte Unpacking "/1
  "Byte Unpacking "/8 -> Data Type Conversion7/1
  "Byte Unpacking "/7 -> Data Type Conversion6/1
  "Byte Unpacking "/5 -> Data Type Conversion4/1
  "Byte Unpacking "/6 -> Data Type Conversion5/1
  Data Type Conversion3/1 -> Gain5/1
  Data Type Conversion4/1 -> Gain6/1
  Data Type Conversion5/1 -> Gain7/1
  Data Type Conversion6/1 -> Gain8/1
  Data Type Conversion7/1 -> Gain9/1
  "Byte Unpacking "/9 -> Data Type Conversion8/1
  Gain4/1 -> X (m)/1
  Data Type Conversion2/1 -> Gain4/1
  Gain5/1 -> Y (m)/1
  Gain6/1 -> Z (m)/1
  Gain7/1 -> alpha (radians)/1
  Gain8/1 -> beta (radians)/1
  Gain9/1 -> gamma (radians)/1
  Data Type Conversion/1 -> Terminator1/1
  Data Type Conversion1/1 -> Terminator2/1
  Data Type Conversion8/1 -> Terminator3/1

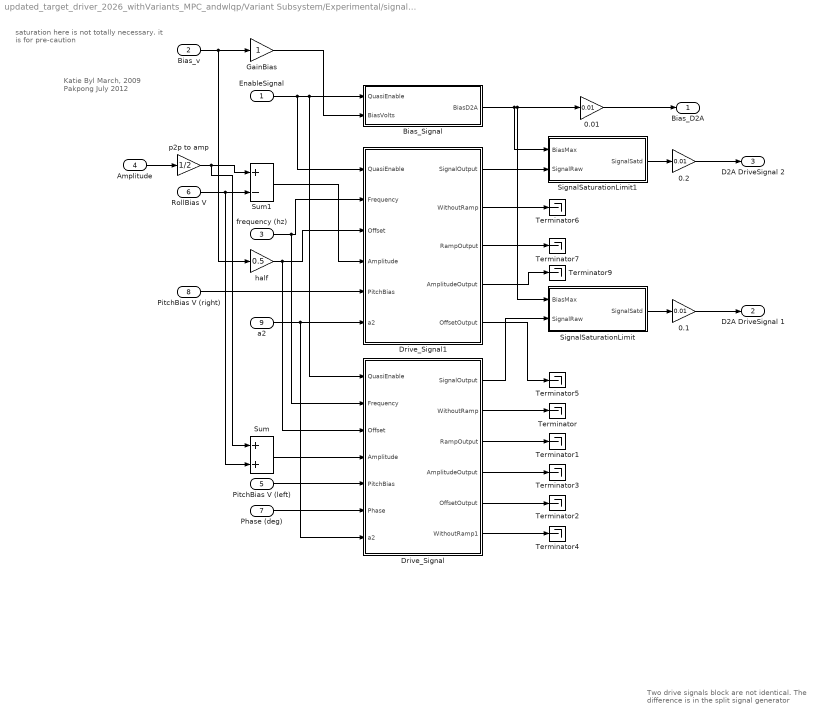
== system updated_target_driver_2026_withVariants_MPC_andwlqp/Variant Subsystem/Experimental/signal generator a3 ==
  note: Katie Byl
      | March, 2009
      |
      | Pakpong
      | July 2012
  note: Two drive signals block are not identical.
      | The difference is in the split signal generator
  note: saturation here is not totally necessary.
      | it is for pre-caution
  EnableSignal : Inport
  Bias_v : Inport  Port=2
  frequency (hz) : Inport  Port=3
  Amplitude : Inport  Port=4
  PitchBias V (left) : Inport  Port=5
  RollBias V : Inport  Port=6
  Phase (deg) : Inport  Port=7
  PitchBias V (right) : Inport  Port=8
  a2 : Inport  Port=9
  0.01 : Gain  Gain=0.01
  0.1 : Gain  Gain=0.01
  0.2 : Gain  Gain=0.01
  Bias_Signal : Subsystem
  Drive_Signal : Subsystem
  Drive_Signal1 : Subsystem
  GainBias : Gain
  SignalSaturationLimit : Subsystem
  SignalSaturationLimit1 : Subsystem
  Sum : Sum
  Sum1 : Sum  Inputs=+-
  Terminator{,1..7,9} (9 alike) : Terminator
  half : Gain  Gain=0.5
  p2p to amp : Gain  Gain=1/2
  Bias_D2A : Outport
  D2A DriveSignal 1 : Outport  Port=2
  D2A DriveSignal 2 : Outport  Port=3
  wires:
  0.1/1 -> D2A DriveSignal 1/1
  0.2/1 -> D2A DriveSignal 2/1
  SignalSaturationLimit1/1(SignalSatd) -> 0.2/1
  0.01/1 -> Bias_D2A/1
  SignalSaturationLimit/1(SignalSatd) -> 0.1/1
  Drive_Signal/5(OffsetOutput) -> Terminator2/1
  GainBias/1 -> Bias_Signal/2(BiasVolts)
  Drive_Signal/1(SignalOutput) -> SignalSaturationLimit/2(SignalRaw)
  Drive_Signal1/5(OffsetOutput) -> Terminator5/1
  half/1 -> Drive_Signal1/3(Offset), Drive_Signal/3(Offset)
  Drive_Signal1/4(AmplitudeOutput) -> Terminator9/1
  Drive_Signal1/3(RampOutput) -> Terminator7/1
  PitchBias V (left)/1 -> Drive_Signal/5(PitchBias)
  Bias_Signal/1(BiasD2A) -> 0.01/1, SignalSaturationLimit/1(BiasMax), SignalSaturationLimit1/1(BiasMax)
  Drive_Signal1/2(WithoutRamp) -> Terminator6/1
  Drive_Signal/6(WithoutRamp1) -> Terminator4/1
  a2/1 -> Drive_Signal1/6(a2), Drive_Signal/7("a2 ")
  Drive_Signal/2(WithoutRamp) -> Terminator/1
  Phase (deg)/1 -> Drive_Signal/6(Phase)
  frequency (hz)/1 -> Drive_Signal/2(Frequency), Drive_Signal1/2(Frequency)
  RollBias V/1 -> Sum1/2, Sum/2
  Sum1/1 -> Drive_Signal1/4(Amplitude)
  Drive_Signal/4(AmplitudeOutput) -> Terminator3/1
  PitchBias V (right)/1 -> Drive_Signal1/5(PitchBias)
  EnableSignal/1 -> Bias_Signal/1(QuasiEnable), Drive_Signal/1(QuasiEnable), Drive_Signal1/1(QuasiEnable)
  Amplitude/1 -> p2p to amp/1
  Sum/1 -> Drive_Signal/4(Amplitude)
  Bias_v/1 -> half/1, GainBias/1
  Drive_Signal/3(RampOutput) -> Terminator1/1
  Drive_Signal1/1(SignalOutput) -> SignalSaturationLimit1/2(SignalRaw)
  p2p to amp/1 -> Sum1/1, Sum/1

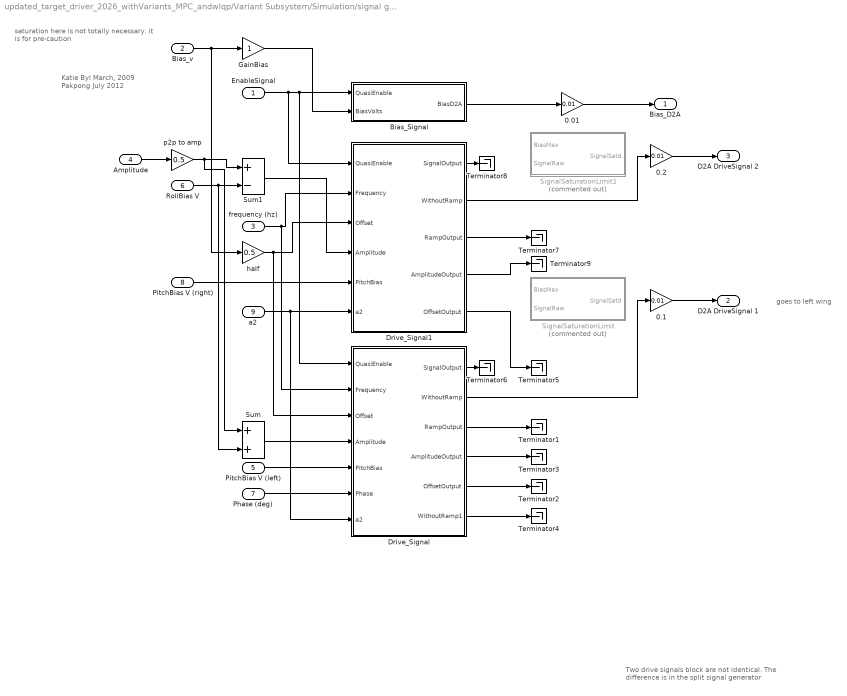
== system updated_target_driver_2026_withVariants_MPC_andwlqp/Variant Subsystem/Simulation/signal generator a3 ==
  note: Katie Byl
      | March, 2009
      |
      | Pakpong
      | July 2012
  note: Two drive signals block are not identical.
      | The difference is in the split signal generator
  note: saturation here is not totally necessary.
      | it is for pre-caution
  note: goes to left wing
  EnableSignal : Inport
  Bias_v : Inport  Port=2
  frequency (hz) : Inport  Port=3
  Amplitude : Inport  Port=4
  PitchBias V (left) : Inport  Port=5
  RollBias V : Inport  Port=6
  Phase (deg) : Inport  Port=7
  PitchBias V (right) : Inport  Port=8
  a2 : Inport  Port=9
  0.01 : Gain  Gain=0.01
  0.1 : Gain  Gain=0.01
  0.2 : Gain  Gain=0.01
  Bias_Signal : Subsystem
  Drive_Signal : Subsystem
  Drive_Signal1 : Subsystem
  GainBias : Gain
  SignalSaturationLimit : Subsystem  Commented=on
  SignalSaturationLimit1 : Subsystem  Commented=on
  Sum : Sum
  Sum1 : Sum  Inputs=+-
  Terminator{1..9} (9 alike) : Terminator
  half : Gain  Gain=0.5
  p2p to amp : Gain  Gain=0.5
  Bias_D2A : Outport
  D2A DriveSignal 1 : Outport  Port=2
  D2A DriveSignal 2 : Outport  Port=3
  wires:
  0.1/1 -> D2A DriveSignal 1/1
  0.2/1 -> D2A DriveSignal 2/1
  0.01/1 -> Bias_D2A/1
  Drive_Signal/5(OffsetOutput) -> Terminator2/1
  GainBias/1 -> Bias_Signal/2(BiasVolts)
  Drive_Signal1/5(OffsetOutput) -> Terminator5/1
  half/1 -> Drive_Signal1/3(Offset), Drive_Signal/3(Offset)
  Drive_Signal1/4(AmplitudeOutput) -> Terminator9/1
  Drive_Signal1/3(RampOutput) -> Terminator7/1
  PitchBias V (left)/1 -> Drive_Signal/5(PitchBias)
  Bias_Signal/1(BiasD2A) -> 0.01/1
  Drive_Signal/6(WithoutRamp1) -> Terminator4/1
  a2/1 -> Drive_Signal1/6(a2), Drive_Signal/7("a2 ")
  Phase (deg)/1 -> Drive_Signal/6(Phase)
  frequency (hz)/1 -> Drive_Signal/2(Frequency), Drive_Signal1/2(Frequency)
  RollBias V/1 -> Sum1/2, Sum/2
  Sum1/1 -> Drive_Signal1/4(Amplitude)
  Drive_Signal/4(AmplitudeOutput) -> Terminator3/1
  PitchBias V (right)/1 -> Drive_Signal1/5(PitchBias)
  EnableSignal/1 -> Bias_Signal/1(QuasiEnable), Drive_Signal/1(QuasiEnable), Drive_Signal1/1(QuasiEnable)
  Amplitude/1 -> p2p to amp/1
  Sum/1 -> Drive_Signal/4(Amplitude)
  Bias_v/1 -> half/1, GainBias/1
  Drive_Signal/3(RampOutput) -> Terminator1/1
  p2p to amp/1 -> Sum1/1, Sum/1
  Drive_Signal1/2(WithoutRamp) -> 0.2/1
  Drive_Signal1/1(SignalOutput) -> Terminator8/1
  Drive_Signal/1(SignalOutput) -> Terminator6/1
  Drive_Signal/2(WithoutRamp) -> 0.1/1

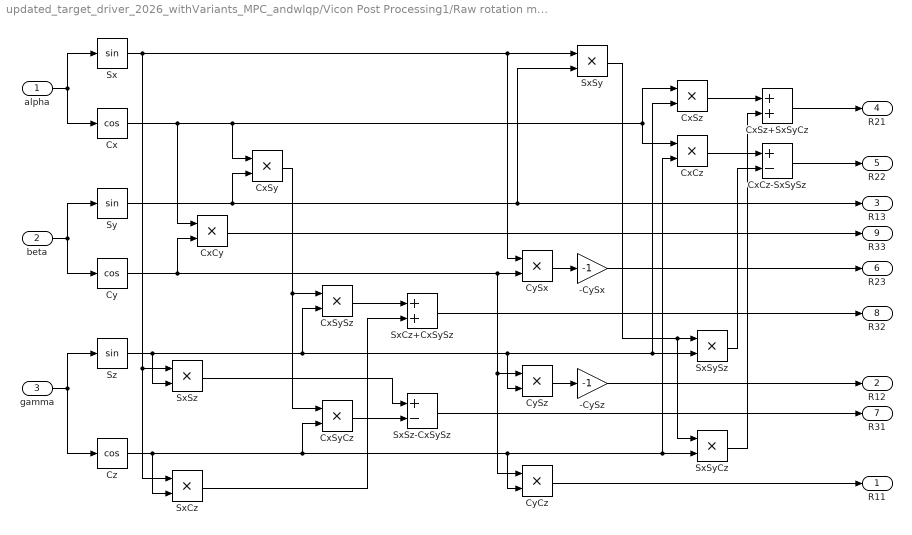
== system updated_target_driver_2026_withVariants_MPC_andwlqp/Vicon Post Processing1/Raw rotation matrix/Rotation Matrix ==
  alpha : Inport
  beta : Inport  Port=2
  gamma : Inport  Port=3
  -CySx : Gain  Gain=-1
  -CySz : Gain  Gain=-1
  Cx : Trigonometry  Operator=cos
  CxCy : Product  RndMeth=Zero
  CxCz : Product  RndMeth=Zero
  CxCz-SxSySz : Sum  Inputs=+-
  CxSy : Product  RndMeth=Zero
  CxSyCz : Product  RndMeth=Zero
  CxSySz : Product  RndMeth=Zero
  CxSz : Product  RndMeth=Zero
  CxSz+SxSyCz : Sum
  Cy : Trigonometry  Operator=cos
  CyCz : Product  RndMeth=Zero
  CySx : Product  RndMeth=Zero
  CySz : Product  RndMeth=Zero
  Cz : Trigonometry  Operator=cos
  Sx : Trigonometry
  SxCz : Product  RndMeth=Zero
  SxCz+CxSySz : Sum
  SxSy : Product  RndMeth=Zero
  SxSyCz : Product  RndMeth=Zero
  SxSySz : Product  RndMeth=Zero
  SxSz : Product  RndMeth=Zero
  SxSz-CxSySz : Sum  Inputs=+-
  Sy : Trigonometry
  Sz : Trigonometry
  R11 : Outport
  R12 : Outport  Port=2
  R13 : Outport  Port=3
  R21 : Outport  Port=4
  R22 : Outport  Port=5
  R23 : Outport  Port=6
  R31 : Outport  Port=7
  R32 : Outport  Port=8
  R33 : Outport  Port=9
  wires:
  beta/1 -> Sy/1, Cy/1
  alpha/1 -> Sx/1, Cx/1
  Sy/1 -> R13/1, SxSy/2, CxSy/2
  Cy/1 -> CySx/2, CySz/1, CyCz/1, CxCy/2
  CySx/1 -> -CySx/1
  -CySx/1 -> R23/1
  gamma/1 -> Sz/1, Cz/1
  Sx/1 -> CySx/1, SxSy/1, SxCz/1, SxSz/1
  SxSy/1 -> SxSyCz/1, SxSySz/1
  Sz/1 -> SxSySz/2, CxSz/2, CySz/2, CxSySz/2, SxSz/2
  Cz/1 -> SxSyCz/2, CxCz/2, CyCz/2, CxSyCz/2, SxCz/2
  Cx/1 -> CxSz/1, CxCz/1, CxSy/1, CxCy/1
  SxSyCz/1 -> CxSz+SxSyCz/2
  CxSz/1 -> CxSz+SxSyCz/1
  CxCz/1 -> CxCz-SxSySz/1
  SxSySz/1 -> CxCz-SxSySz/2
  CySz/1 -> -CySz/1
  CyCz/1 -> R11/1
  -CySz/1 -> R12/1
  CxSz+SxSyCz/1 -> R21/1
  CxCz-SxSySz/1 -> R22/1
  CxSy/1 -> CxSySz/1, CxSyCz/1
  CxSySz/1 -> SxCz+CxSySz/1
  SxCz/1 -> SxCz+CxSySz/2
  CxSyCz/1 -> SxSz-CxSySz/2
  SxSz/1 -> SxSz-CxSySz/1
  SxSz-CxSySz/1 -> R31/1
  SxCz+CxSySz/1 -> R32/1
  CxCy/1 -> R33/1

== system updated_target_driver_2026_withVariants_MPC_andwlqp/Vicon Post Processing1/Vicon Validity check/Variant Subsystem1 ==
  note: 1) Add Subsystem or Model blocks as valid variant choices.
      | 2) You cannot connect blocks at this level. At simulation, connectivity is automatically
      | determined, based on the active variant and port name matching.
  In1 : Inport
  Experimental : Subsystem  VariantControl=Plant==1
  Simulation : Subsystem  VariantControl=Plant==2
  Out1 : Outport

== system updated_target_driver_2026_withVariants_MPC_andwlqp/Desired attitude and normalized error/Variant Subsystem/saturated normalized error observation/Saturated angular velocity eOmega  ==
  omega : Inport
  "omega_desired " : Inport  Port=2
  R_cur : Inport  Port=3
  R_desired : Inport  Port=4
  Compute attitude error eR : MATLAB Function  TreatAsAtomicUnit=on
  Demux1 : Demux  Outputs=3
  Gain : Gain  Gain=2/(upp_bound-low_bound)
  Gain1 : Gain  Gain=2/(upp_bound-low_bound)
  Gain2 : Gain  Gain=2/(upp_bound-low_bound)
  Mux5 : Mux  Inputs=3
  Saturation1 : Saturate  UpperLimit=upp_bound  LowerLimit=low_bound
  Saturation2 : Saturate  UpperLimit=upp_bound  LowerLimit=low_bound
  Saturation3 : Saturate  UpperLimit=upp_bound  LowerLimit=low_bound
  Normalized angular velocity : Outport
  wires:
  Saturation1/1 -> Gain/1
  Mux5/1 -> Normalized angular velocity/1
  Saturation2/1 -> Gain1/1
  Gain/1 -> Mux5/1
  Gain1/1 -> Mux5/2
  "omega_desired "/1 -> Compute attitude error eR/4(omega_desired)
  Demux1/1 -> Saturation1/1
  R_desired/1 -> Compute attitude error eR/2(R_desired)
  R_cur/1 -> Compute attitude error eR/1(R_cur)
  omega/1 -> Compute attitude error eR/3(omega)
  Compute attitude error eR/1(y) -> Demux1/1
  Demux1/2 -> Saturation2/1
  Demux1/3 -> Saturation3/1
  Saturation3/1 -> Gain2/1
  Gain2/1 -> Mux5/3

== system updated_target_driver_2026_withVariants_MPC_andwlqp/Desired attitude and normalized error/Variant Subsystem/saturated normalized error observation/Saturated normalized eR ==
  Current averaged rotation M : Inport
  R_desired : Inport  Port=2
  Compute attitude error eR : MATLAB Function  TreatAsAtomicUnit=on
  Gain6 : Gain  Gain=2/(upp_bound_eR-low_bound_eR)
  Saturation4 : Saturate  UpperLimit=upp_bound_eR  LowerLimit=low_bound_eR
  normalized eR : Outport
  wires:
  Compute attitude error eR/1(y) -> Saturation4/1
  Saturation4/1 -> Gain6/1
  R_desired/1 -> Compute attitude error eR/2(R_desired)
  Gain6/1 -> normalized eR/1
  Current averaged rotation M/1 -> Compute attitude error eR/1(R_cur)

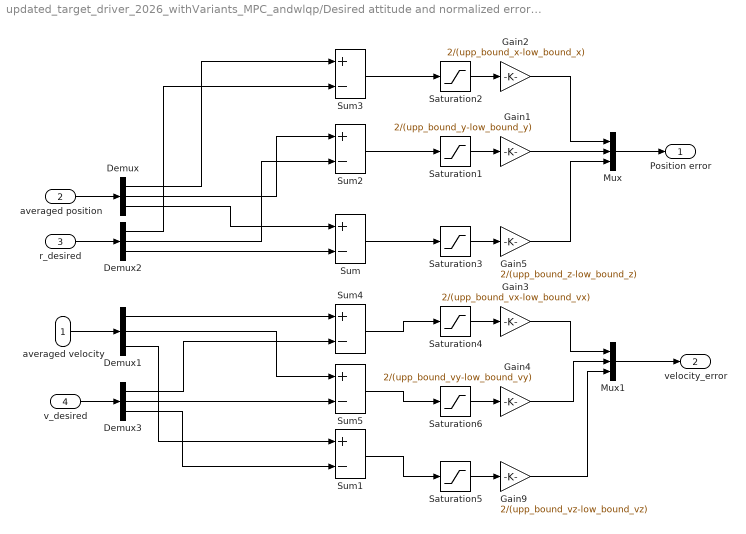
== system updated_target_driver_2026_withVariants_MPC_andwlqp/Desired attitude and normalized error/Variant Subsystem/saturated normalized error observation/saturated normalized altitude error  ==
  averaged velocity : Inport
  averaged position : Inport  Port=2
  "r_desired " : Inport  Port=3
  v_desired : Inport  Port=4
  Demux{,1..3} (4 alike) : Demux  Outputs=3
  Gain1 : Gain  Gain=2/(upp_bound_y-low_bound_y)
  Gain2 : Gain  Gain=2/(upp_bound_x-low_bound_x)
  Gain3 : Gain  Gain=2/(upp_bound_vx-low_bound_vx)
  Gain4 : Gain  Gain=2/(upp_bound_vy-low_bound_vy)
  Gain5 : Gain  Gain=2/(upp_bound_z-low_bound_z)
  Gain9 : Gain  Gain=2/(upp_bound_vz-low_bound_vz)
  Mux : Mux  Inputs=3
  Mux1 : Mux  Inputs=3
  Saturation1 : Saturate  UpperLimit=upp_bound_y  LowerLimit=low_bound_y
  Saturation2 : Saturate  UpperLimit=upp_bound_x  LowerLimit=low_bound_x
  Saturation3 : Saturate  UpperLimit=upp_bound_z  LowerLimit=low_bound_z
  Saturation4 : Saturate  UpperLimit=upp_bound_vx  LowerLimit=low_bound_vx
  Saturation5 : Saturate  UpperLimit=upp_bound_vz  LowerLimit=low_bound_vz
  Saturation6 : Saturate  UpperLimit=upp_bound_vy  LowerLimit=low_bound_vy
  Sum{,1..5} (6 alike) : Sum  Inputs=+-
  Position error : Outport
  velocity_error : Outport  Port=2
  wires:
  Demux2/3 -> Sum/2
  Sum/1 -> Saturation3/1
  Sum1/1 -> Saturation5/1
  Gain5/1 -> Mux/3
  Saturation3/1 -> Gain5/1
  Saturation5/1 -> Gain9/1
  Gain9/1 -> Mux1/3
  Mux1/1 -> velocity_error/1
  averaged velocity/1 -> Demux1/1
  averaged position/1 -> Demux/1
  Demux/3 -> Sum/1
  Demux1/3 -> Sum1/1
  "r_desired "/1 -> Demux2/1
  Saturation1/1 -> Gain1/1
  Sum2/1 -> Saturation1/1
  Demux2/2 -> Sum2/2
  Demux/2 -> Sum2/1
  Sum3/1 -> Saturation2/1
  Saturation2/1 -> Gain2/1
  Demux/1 -> Sum3/1
  Demux2/1 -> Sum3/2
  v_desired/1 -> Demux3/1
  Demux3/3 -> Sum1/2
  Saturation4/1 -> Gain3/1
  Gain3/1 -> Mux1/1
  Sum4/1 -> Saturation4/1
  Demux3/1 -> Sum4/2
  Demux1/1 -> Sum4/1
  Saturation6/1 -> Gain4/1
  Gain4/1 -> Mux1/2
  Sum5/1 -> Saturation6/1
  Demux3/2 -> Sum5/2
  Demux1/2 -> Sum5/1
  Gain2/1 -> Mux/1
  Gain1/1 -> Mux/2
  Mux/1 -> Position error/1

== system updated_target_driver_2026_withVariants_MPC_andwlqp/Desired attitude and normalized error/Variant Subsystem/unsaturated normalized error observation1/Saturated angular velocity eOmega  ==
  omega : Inport
  "omega_desired " : Inport  Port=2
  R_cur : Inport  Port=3
  R_desired : Inport  Port=4
  Compute attitude error eR : MATLAB Function  TreatAsAtomicUnit=on
  Demux1 : Demux  Outputs=3
  Gain : Gain  Commented=through  Gain=2/(upp_bound-low_bound)
  Gain1 : Gain  Commented=through  Gain=2/(upp_bound-low_bound)
  Gain2 : Gain  Commented=through  Gain=2/(upp_bound-low_bound)
  Mux5 : Mux  Inputs=3
  Saturation1 : Saturate  Commented=through  UpperLimit=upp_bound  LowerLimit=low_bound
  Saturation2 : Saturate  Commented=through  UpperLimit=upp_bound  LowerLimit=low_bound
  Saturation3 : Saturate  Commented=through  UpperLimit=upp_bound  LowerLimit=low_bound
  Normalized angular velocity : Outport
  wires:
  Saturation1/1 -> Gain/1
  Mux5/1 -> Normalized angular velocity/1
  Saturation2/1 -> Gain1/1
  Gain/1 -> Mux5/1
  Gain1/1 -> Mux5/2
  "omega_desired "/1 -> Compute attitude error eR/4(omega_desired)
  Demux1/1 -> Saturation1/1
  R_desired/1 -> Compute attitude error eR/2(R_desired)
  R_cur/1 -> Compute attitude error eR/1(R_cur)
  omega/1 -> Compute attitude error eR/3(omega)
  Compute attitude error eR/1(y) -> Demux1/1
  Demux1/2 -> Saturation2/1
  Demux1/3 -> Saturation3/1
  Saturation3/1 -> Gain2/1
  Gain2/1 -> Mux5/3

== system updated_target_driver_2026_withVariants_MPC_andwlqp/Desired attitude and normalized error/Variant Subsystem/unsaturated normalized error observation1/Saturated normalized eR ==
  Current averaged rotation M : Inport
  R_desired : Inport  Port=2
  Compute attitude error eR : MATLAB Function  TreatAsAtomicUnit=on
  Gain6 : Gain  Commented=through  Gain=2/(upp_bound_eR-low_bound_eR)
  Saturation4 : Saturate  Commented=through  UpperLimit=upp_bound_eR  LowerLimit=low_bound_eR
  normalized eR : Outport
  wires:
  Compute attitude error eR/1(y) -> Saturation4/1
  Saturation4/1 -> Gain6/1
  R_desired/1 -> Compute attitude error eR/2(R_desired)
  Gain6/1 -> normalized eR/1
  Current averaged rotation M/1 -> Compute attitude error eR/1(R_cur)
